simulink model "Battery_TempPredUsingNN_PhysicsModel"  (R2020b)
settings: Solver=ode1be  StartTime=0.0  StopTime=4000  FixedStep=1  MaxStep=5e-2  RelTol=1e-3  AbsTol=1e-3
PreLoadFcn:
  | Battery_TempPredUsingNN_PhysicsModel_ini
undefined symbols (not defined in the file): ambient, Flowrate_vec, FlwR, FlwT
libraries: nesl_utility x19, fl_lib x9, batteryModule_lib x4
Description:
  | Battery Pack Plant Model For Training Neural Network
settings Model: Creator=The MathWorks, Inc.  LastModifiedBy=vikrants
settings SolverCC: AutoScaleAbsTol=off  ZeroCrossAlgorithm=Adaptive
settings DataIOCC: ReturnWorkspaceOutputs=off
settings DebuggingCC: IgnoredZcDiagnostic=none  SymbolicDimsDataTypeCodeGenerationDiagnostic=none
settings SFSimCC: CustomCodeUndefinedFunction=UseInterfaceOnly
settings SimscapeCC: SimscapeLogType=all  SimscapeLogSimulationStatistics=on  SimscapeLogName=simlog_Battery_TempPredUsingNN_PhysicsModel  SimscapeLogDataHistory=250000

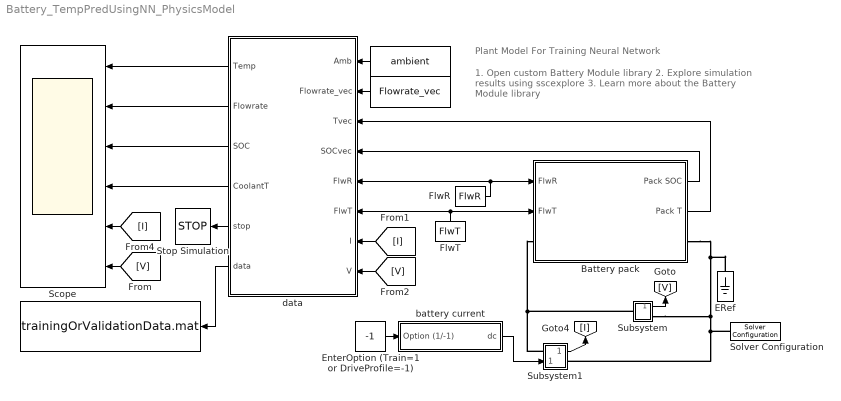
== system Battery_TempPredUsingNN_PhysicsModel ==
  note: Plant Model For Training Neural Network
  note: 1. Open custom Battery Module library
      | 2. Explore simulation results using sscexplore
      | 3. Learn more about the Battery Module library
  " " : ToFile  Filename=trainingOrValidationData.mat  MatrixName=validate_X  SaveFormat=Timeseries
  "    " : Constant  Value=Flowrate_vec
  "       " : Constant  Value=ambient
  Battery pack : Subsystem
      mask Display: image('Battery_Management_System_icon.png'); % Use "Edit Image" on toolstrip to change.
  "ERef " : fl_lib/Electrical/Electrical Elements/Electrical Reference
  EnterOption (Train=1 or DriveProfile=-1) : Constant  Value=-1
  FlwR : Constant  Value=FlwR
  FlwT : Constant  Value=FlwT
  Scope : Scope  NumInputPorts=6
  Solver Configuration : nesl_utility/Solver Configuration  PhysicalDomain=network_engine_domain  SubClassName=solver  LeftPortType=input  RightPortType=generic  Tones=[]  Harmonics=[]  SimulateNoise=off  Profile=off  UseLocalSampling=off  EnableSwitchedLinearOptims=on  FrequencyDomain=off  UseCCode=off  RelTol=0.001  AbsTol=1e-06  MinStep=1e-09  ToWorkspace=off  RevertToSquareIcSolve=off  NumHomotopyIterations=100  PhasorMode=off  PhasorModeNumHarmonics=1  DoDC=off  ResidualTolerance=1e-09  UseLocalSolver=on  LocalSolverChoice=NE_BACKWARD_EULER_ADVANCER  LocalSolverSampleTime=1  DoFixedCost=on  MaxNonlinIter=3  MaxModeIter=2  ComputeImpulses=off  ImpulseIterations=1  LinearAlgebra=auto  EquationFormulation=NE_TIME_EF  DelaysMemoryBudget=1024  AutomaticFiltering=on  FilteringTimeConstant=0.001  PartitionStorageMethod=AS_NEEDED  PartitionMemoryBudget=1024  PartitionMethod=ROBUST
      settings: SourceProductBaseCode=PW,SS
  Stop Simulation : Stop
  Subsystem : Subsystem
  Subsystem1 : Subsystem
      settings: PortSchema="{\"entries\":[{\"content\":{\"sides\":[{\"content\":{\"connectorIds\":[\"LConn1\",\"In1\"]},\"type\":\"ConnectorPlacement.EquallySpacedRectSide\",\"uuid\":\"67d2af16-eb6a-4131-a21a-c97dc5606bfb\"},{\"content\":{\"connectorIds\":[\"Out1\",\"RConn1\"],\"side\":\"RIGHT\"},\"type\":\"ConnectorPlacement.EquallySpacedRectSide\",\"uuid\":\"35a4b5c9-72e5-421e-bb7c-ed2a1ed376d5\"},{\"content\":{\"connectorIds\":[],\"side\":\"TOP\"},\"type\":\"ConnectorPlacement.EquallySpacedRectSide\",\"uuid\":\"8dbff2ba-7191-4b7c-8c3d-553f583a3f33\"},{\"content\":{\"connectorIds\":[],\"side\":\"HIDDEN\"},\"type\":\"ConnectorPlacement.EquallySpacedRectSide\",\"uuid\":\"d4ede02e-0aa1-49c8-8ab9-b8bb5b8f4755\"}]},\"type\":\"ConnectorPlacement.EquallySpacedConnector\",\"uuid\":\"f2085621-9cc2-4a00-8d4f-41f8dda0152d\"}],\"packageUris\":[\"http://schema.mathworks.com/mf0/Connector/R2020b\"],\"version\":\"1.0\"}"
  battery current : Subsystem
  data : Subsystem
  wires:
  Battery pack/2(Pack T) -> data/3(Tvec)
  Battery pack/1(Pack SOC) -> data/4(SOCvec)
  "    "/1 -> data/2(Flowrate_vec)
  "       "/1 -> data/1(Amb)
  [I] -> Scope/5
  data/3(SOC) -> Scope/3
  data/2(Flowrate) -> Scope/2
  FlwT/1 -> data/6(FlwT), Battery pack/2(FlwT)
  data/4(CoolantT) -> Scope/4
  [V] -> Scope/6
  [I] -> data/7(I)
  data/5(stop) -> Stop Simulation/1
  data/6(data) -> " "/1
  [V] -> data/8(V)
  data/1(Temp) -> Scope/1
  FlwR/1 -> Battery pack/1(FlwR), data/5(FlwR)
  Subsystem/1("   ") -> [V]
  Subsystem1/1("   ") -> [I]
  EnterOption (Train=1 or DriveProfile=-1)/1 -> battery current/1(Option (1/-1))
  battery current/1(dc) -> Subsystem1/1(dc)
  connections:
  Battery pack/RConn1 -- "ERef "/LConn1 -- Solver Configuration/RConn1 -- Subsystem1/RConn1 -- Subsystem/RConn1
  Subsystem/LConn1 -- Subsystem1/LConn1 -- Battery pack/LConn1

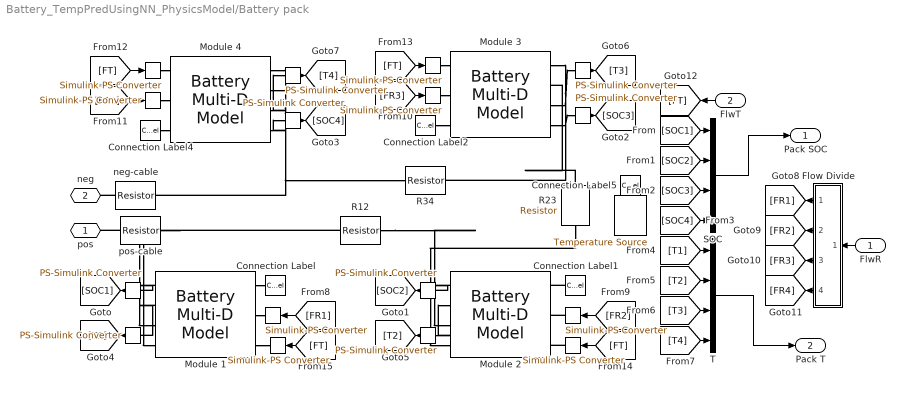
== system Battery_TempPredUsingNN_PhysicsModel/Battery pack ==
  FlwR : Inport
  FlwT : Inport  Port=2
  " " : nesl_utility/PS-Simulink Converter  PhysicalDomain=network_engine_domain  SubClassName=ps_output  LeftPortType=input  RightPortType=output  PseudoPeriodic=off  Frequencies=[]  Unit=inherit  AffineConversion=off
      settings: SourceProductBaseCode=PW,SS
  "  " : nesl_utility/PS-Simulink Converter  PhysicalDomain=network_engine_domain  SubClassName=ps_output  LeftPortType=input  RightPortType=output  PseudoPeriodic=off  Frequencies=[]  Unit=inherit  AffineConversion=off
      settings: SourceProductBaseCode=PW,SS
  "   " : nesl_utility/PS-Simulink Converter  PhysicalDomain=network_engine_domain  SubClassName=ps_output  LeftPortType=input  RightPortType=output  PseudoPeriodic=off  Frequencies=[]  Unit=inherit  AffineConversion=off
      settings: SourceProductBaseCode=PW,SS
  "    " : nesl_utility/Simulink-PS Converter  PhysicalDomain=network_engine_domain  SubClassName=ps_input  LeftPortType=input  RightPortType=output  PseudoPeriodic=off  Frequencies=[]  NoiseDistribution=none  NoiseParameters=[]  Unit=1  AffineConversion=off  FilteringAndDerivatives=filter  SimscapeFilterOrder=1  InputFilterTimeConstant=0.01  UdotUserProvided=0
      settings: SourceProductBaseCode=PW,SS
  "     " : fl_lib/Thermal/Thermal Sources/Temperature Source  temperature=ambient K
  "      " : nesl_utility/PS-Simulink Converter  PhysicalDomain=network_engine_domain  SubClassName=ps_output  LeftPortType=input  RightPortType=output  PseudoPeriodic=off  Frequencies=[]  Unit=inherit  AffineConversion=off
      settings: SourceProductBaseCode=PW,SS
  "       " : nesl_utility/Simulink-PS Converter  PhysicalDomain=network_engine_domain  SubClassName=ps_input  LeftPortType=input  RightPortType=output  PseudoPeriodic=off  Frequencies=[]  NoiseDistribution=none  NoiseParameters=[]  Unit=1  AffineConversion=off  FilteringAndDerivatives=filter  SimscapeFilterOrder=1  InputFilterTimeConstant=0.01  UdotUserProvided=0
      settings: SourceProductBaseCode=PW,SS
  "         " : nesl_utility/PS-Simulink Converter  PhysicalDomain=network_engine_domain  SubClassName=ps_output  LeftPortType=input  RightPortType=output  PseudoPeriodic=off  Frequencies=[]  Unit=inherit  AffineConversion=off
      settings: SourceProductBaseCode=PW,SS
  "          " : nesl_utility/PS-Simulink Converter  PhysicalDomain=network_engine_domain  SubClassName=ps_output  LeftPortType=input  RightPortType=output  PseudoPeriodic=off  Frequencies=[]  Unit=inherit  AffineConversion=off
      settings: SourceProductBaseCode=PW,SS
  "           " : nesl_utility/Simulink-PS Converter  PhysicalDomain=network_engine_domain  SubClassName=ps_input  LeftPortType=input  RightPortType=output  PseudoPeriodic=off  Frequencies=[]  NoiseDistribution=none  NoiseParameters=[]  Unit=1  AffineConversion=off  FilteringAndDerivatives=filter  SimscapeFilterOrder=1  InputFilterTimeConstant=0.01  UdotUserProvided=0
      settings: SourceProductBaseCode=PW,SS
  "            " : nesl_utility/PS-Simulink Converter  PhysicalDomain=network_engine_domain  SubClassName=ps_output  LeftPortType=input  RightPortType=output  PseudoPeriodic=off  Frequencies=[]  Unit=inherit  AffineConversion=off
      settings: SourceProductBaseCode=PW,SS
  "              " : nesl_utility/Simulink-PS Converter  PhysicalDomain=network_engine_domain  SubClassName=ps_input  LeftPortType=input  RightPortType=output  PseudoPeriodic=off  Frequencies=[]  NoiseDistribution=none  NoiseParameters=[]  Unit=1  AffineConversion=off  FilteringAndDerivatives=filter  SimscapeFilterOrder=1  InputFilterTimeConstant=0.01  UdotUserProvided=0
      settings: SourceProductBaseCode=PW,SS
  "               " : nesl_utility/Simulink-PS Converter  PhysicalDomain=network_engine_domain  SubClassName=ps_input  LeftPortType=input  RightPortType=output  PseudoPeriodic=off  Frequencies=[]  NoiseDistribution=none  NoiseParameters=[]  Unit=1  AffineConversion=off  FilteringAndDerivatives=filter  SimscapeFilterOrder=1  InputFilterTimeConstant=0.01  UdotUserProvided=0
      settings: SourceProductBaseCode=PW,SS
  "                      " : nesl_utility/Simulink-PS Converter  PhysicalDomain=network_engine_domain  SubClassName=ps_input  LeftPortType=input  RightPortType=output  PseudoPeriodic=off  Frequencies=[]  NoiseDistribution=none  NoiseParameters=[]  Unit=1  AffineConversion=off  FilteringAndDerivatives=filter  SimscapeFilterOrder=1  InputFilterTimeConstant=0.01  UdotUserProvided=0
      settings: SourceProductBaseCode=PW,SS
  "                                      " : nesl_utility/PS-Simulink Converter  PhysicalDomain=network_engine_domain  SubClassName=ps_output  LeftPortType=input  RightPortType=output  PseudoPeriodic=off  Frequencies=[]  Unit=inherit  AffineConversion=off
      settings: SourceProductBaseCode=PW,SS
  "                                           " : nesl_utility/Simulink-PS Converter  PhysicalDomain=network_engine_domain  SubClassName=ps_input  LeftPortType=input  RightPortType=output  PseudoPeriodic=off  Frequencies=[]  NoiseDistribution=none  NoiseParameters=[]  Unit=1  AffineConversion=off  FilteringAndDerivatives=filter  SimscapeFilterOrder=1  InputFilterTimeConstant=0.01  UdotUserProvided=0
      settings: SourceProductBaseCode=PW,SS
  "                                                  " : nesl_utility/Simulink-PS Converter  PhysicalDomain=network_engine_domain  SubClassName=ps_input  LeftPortType=input  RightPortType=output  PseudoPeriodic=off  Frequencies=[]  NoiseDistribution=none  NoiseParameters=[]  Unit=1  AffineConversion=off  FilteringAndDerivatives=filter  SimscapeFilterOrder=1  InputFilterTimeConstant=0.01  UdotUserProvided=0
      settings: SourceProductBaseCode=PW,SS
  "                        Flow Divide" : Subsystem
  Connection Label{,1..2,4..5} (5 alike) : ConnectionLabel  Label=Amb
  Module 1 : batteryModule_lib/Battery Multi-D Model  modelComplexity=batteryModule.batteryAbstractionLevel.detailed  thermalManagement=batteryModule.batteryCoolingSystem.thermalPort  thermal_moduleBottom=batteryModule.batteryThermalPortSelection.thermalLUT  thermal_moduleTop=batteryModule.batteryThermalPortSelection.convectionBC  thermal_moduleLeft=batteryModule.batteryThermalPortSelection.convectionBC  thermal_moduleRight=batteryModule.batteryThermalPortSelection.convectionBC  thermal_modulePos=batteryModule.batteryThermalPortSelection.convectionBC  thermal_moduleNeg=batteryModule.batteryThermalPortSelection.convectionBC  Ns=Ns  Np=Np  cellTypeSelection=batteryModule.batteryTypeSelection.pouch  cellHeight=cell_H m  cellWidth=cell_W m  cellThickness=cell_T m  cellDiameter=0.018 m  cellCylinLine=3  moduleExternalR=Rext Ohm  LUTpointsTemp=T_vec K  LUTpointsSOC=SOC_vec  cellAHvector=AH_vec hr*A  moduleCellAHpercentVar=AhrVar  cellThermalMass=MdotCp J/K  cellThermalCond=K_cell W/(m*K)  cellThermalCond_inPlane=K_cell W/(m*K)  cellHeatTrCoeff=1 W/(m^2 * K)  htc_bottom=1 W/(m^2 * K)  htc_top=h_cell W/(m^2 * K)  htc_right=h_cell W/(m^2 * K)  htc_left=h_cell W/(m^2 * K)  htc_pos=h_cell W/(m^2 * K)  htc_neg=h_cell W/(m^2 * K)  cellTemp=cellT_ini K  cellSOC=cellSOC_ini  LUTpointsFlowrate_b=Flowrate_vec kg/s  LUTpointsTemp_b=T_vec K  LUTpointsFlowrate_t=[.01, .02, .03, .04, .05, .06] kg/s  LUTpointsTemp_t=[273.15, 298.15, 323.15] K  LUTpointsFlowrate_r=[.01, .02, .03, .04, .05, .06] kg/s  LUTpointsTemp_r=[273.15, 298.15, 323.15] K  LUTpointsFlowrate_l=[.01, .02, .03, .04, .05, .06] kg/s  LUTpointsTemp_l=[273.15, 298.15, 323.15] K  LUTpointsFlowrate_p=[.01, .02, .03, .04, .05, .06] kg/s  LUTpointsTemp_p=[273.15, 298.15, 323.15] K  LUTpointsFlowrate_n=[.01, .02, .03, .04, .05, .06] kg/s  LUTpointsTemp_n=[273.15, 298.15, 323.15] K  moduleCooling_b=coolantQ W/K  moduleCooling_t=zeros(3, 6, 10) W/K  moduleCooling_r=zeros(3, 6, 10) W/K  moduleCooling_l=zeros(3, 6, 10) W/K  moduleCooling_p=zeros(3, 6, 10) W/K  moduleCooling_n=zeros(3, 6, 10) W/K  moduleExtHeat=extHeat W  moduleCellBalancing=batteryModule.batteryCellBalancing.none  moduleCellVoltages=batteryModule.batteryCellVoltages.no  passiveShuntR=50 Ohm  passiveSWclosedR=0.01 Ohm  passiveSWopenCond=1e-8 1/Ohm  passiveSWthreshold=0.5  prm_dir=ee.enum.battery.prm_dir.noCurrentDirectionality  V0_mat=V0_mat V  R0_mat=R0_mat Ohm  R0_dis_mat=[.03, .015, .002; .04, .017, .008; .039, .012, .006; .027, .013, .021] Ohm  R0_ch_mat=[.03, .015, .002; .04, .017, .008; .039, .012, .006; .027, .013, .021] Ohm  moduleCellR0PercentVar=R0Var  prm_leak=ee.enum.battery.prm_leak.disabled  Rleak_vec=[8000, 7000, 6000] Ohm  moduleCellLeakPercentVar=ones(1, 10)  extrapolation_option=ee.enum.extrapolation.nearest  prm_dyn=ee.enum.battery.prm_dyn.off  R1_mat=[.089, .076, .01; .042, .022, .099; .019, .007, .002; .051, .043, .029] Ohm  tau1_mat=[44, 148, 235; 93, 110, 1000; 19, 27, 133; .5, 22, 3] s  R2_mat=[.014, .382, .407; .028, .006, .007; .014, .007, .006; .333, .956, .912] Ohm  tau2_mat=[1, 44, 5644; 11, 24, 506; 2, 14, 330; 3310, 13419, 30216] s  R3_mat=[.014, .382, .407; .028, .006, .007; .014, .007, .006; .333, .956, .912] Ohm  tau3_mat=[1, 44, 5644; 11, 24, 506; 2, 14, 330; 3310, 13419, 30216] s  R4_mat=[.014, .382, .407; .028, .006, .007; .014, .007, .006; .333, .956, .912] Ohm  tau4_mat=[1, 44, 5644; 11, 24, 506; 2, 14, 330; 3310, 13419, 30216] s  R5_mat=[.014, .382, .407; .028, .006, .007; .014, .007, .006; .333, .956, .912] Ohm  tau5_mat=[1, 44, 5644; 11, 24, 506; 2, 14, 330; 3310, 13419, 30216] s  prm_fade=ee.enum.battery.prm_fade.equations  N0=Ndisc  dV0=delV0  dR0=delR0  dAH=delAH  dRleak=0  dR1=0  dR2=0  dR3=0  dR4=0  dR5=0  N0vec=[100, 200, 300]  Tfadevec=[298.15, 323.15] K  dV0vec=[0, 0, 0]  dR0vec=[0, 0, 0]  dAHvec=[0, 0, 0]  dRleakvec=[0, 0, 0]  dR1vec=[0, 0, 0]  dR2vec=[0, 0, 0]  dR3vec=[0, 0, 0]  dR4vec=[0, 0, 0]  dR5vec=[0, 0, 0]  dV0mat=[0, 0; 0, 0; 0, 0]  dR0mat=[0, 0; 0, 0; 0, 0]  dAHmat=[0, 0; 0, 0; 0, 0]  dRleakmat=[0, 0; 0, 0; 0, 0]  dR1mat=[0, 0; 0, 0; 0, 0]  dR2mat=[0, 0; 0, 0; 0, 0]  dR3mat=[0, 0; 0, 0; 0, 0]  dR4mat=[0, 0; 0, 0; 0, 0]  dR5mat=[0, 0; 0, 0; 0, 0]
      settings: InternalSimscapePortConfiguration="{\"Bottom\":[],\"Left\":[{\"id\":\"outputCellSOC\",\"label\":\"SOC\",\"type\":\"output\"},{\"id\":\"outputCellTemp\",\"label\":\"Temp\",\"type\":\"output\"}],\"Right\":[{\"id\":\"H\",\"label\":\"Amb\",\"type\":\"foundation.thermal.thermal\"},{\"id\":\"frac_b\",\"label\":\"FlwR\",\"type\":\"input\"},{\"id\":\"delT_b\",\"label\":\"FlwT\",\"type\":\"input\"}],\"Top\":[{\"id\":\"p\",\"label\":\"pos\",\"type\":\"foundation.electrical.electrical\"},{\"id\":\"n\",\"label\":\"neg\",\"type\":\"foundation.electrical.electrical\"}]}"
  Module 2 : batteryModule_lib/Battery Multi-D Model  modelComplexity=batteryModule.batteryAbstractionLevel.detailed  thermalManagement=batteryModule.batteryCoolingSystem.thermalPort  thermal_moduleBottom=batteryModule.batteryThermalPortSelection.thermalLUT  thermal_moduleTop=batteryModule.batteryThermalPortSelection.convectionBC  thermal_moduleLeft=batteryModule.batteryThermalPortSelection.convectionBC  thermal_moduleRight=batteryModule.batteryThermalPortSelection.convectionBC  thermal_modulePos=batteryModule.batteryThermalPortSelection.convectionBC  thermal_moduleNeg=batteryModule.batteryThermalPortSelection.convectionBC  Ns=Ns  Np=Np  cellTypeSelection=batteryModule.batteryTypeSelection.pouch  cellHeight=cell_H m  cellWidth=cell_W m  cellThickness=cell_T m  cellDiameter=0.018 m  cellCylinLine=3  moduleExternalR=Rext Ohm  LUTpointsTemp=T_vec K  LUTpointsSOC=SOC_vec  cellAHvector=AH_vec hr*A  moduleCellAHpercentVar=AhrVar  cellThermalMass=MdotCp J/K  cellThermalCond=K_cell W/(m*K)  cellThermalCond_inPlane=K_cell W/(m*K)  cellHeatTrCoeff=1 W/(m^2 * K)  htc_bottom=1 W/(m^2 * K)  htc_top=h_cell W/(m^2 * K)  htc_right=h_cell W/(m^2 * K)  htc_left=h_cell W/(m^2 * K)  htc_pos=h_cell W/(m^2 * K)  htc_neg=h_cell W/(m^2 * K)  cellTemp=cellT_ini K  cellSOC=cellSOC_ini  LUTpointsFlowrate_b=Flowrate_vec kg/s  LUTpointsTemp_b=T_vec K  LUTpointsFlowrate_t=[.01, .02, .03, .04, .05, .06] kg/s  LUTpointsTemp_t=[273.15, 298.15, 323.15] K  LUTpointsFlowrate_r=[.01, .02, .03, .04, .05, .06] kg/s  LUTpointsTemp_r=[273.15, 298.15, 323.15] K  LUTpointsFlowrate_l=[.01, .02, .03, .04, .05, .06] kg/s  LUTpointsTemp_l=[273.15, 298.15, 323.15] K  LUTpointsFlowrate_p=[.01, .02, .03, .04, .05, .06] kg/s  LUTpointsTemp_p=[273.15, 298.15, 323.15] K  LUTpointsFlowrate_n=[.01, .02, .03, .04, .05, .06] kg/s  LUTpointsTemp_n=[273.15, 298.15, 323.15] K  moduleCooling_b=coolantQ W/K  moduleCooling_t=zeros(3, 6, 10) W/K  moduleCooling_r=zeros(3, 6, 10) W/K  moduleCooling_l=zeros(3, 6, 10) W/K  moduleCooling_p=zeros(3, 6, 10) W/K  moduleCooling_n=zeros(3, 6, 10) W/K  moduleExtHeat=extHeat W  moduleCellBalancing=batteryModule.batteryCellBalancing.none  moduleCellVoltages=batteryModule.batteryCellVoltages.no  passiveShuntR=50 Ohm  passiveSWclosedR=0.01 Ohm  passiveSWopenCond=1e-8 1/Ohm  passiveSWthreshold=0.5  prm_dir=ee.enum.battery.prm_dir.noCurrentDirectionality  V0_mat=V0_mat V  R0_mat=R0_mat Ohm  R0_dis_mat=[.03, .015, .002; .04, .017, .008; .039, .012, .006; .027, .013, .021] Ohm  R0_ch_mat=[.03, .015, .002; .04, .017, .008; .039, .012, .006; .027, .013, .021] Ohm  moduleCellR0PercentVar=R0Var  prm_leak=ee.enum.battery.prm_leak.disabled  Rleak_vec=[8000, 7000, 6000] Ohm  moduleCellLeakPercentVar=ones(1, 10)  extrapolation_option=ee.enum.extrapolation.nearest  prm_dyn=ee.enum.battery.prm_dyn.off  R1_mat=[.089, .076, .01; .042, .022, .099; .019, .007, .002; .051, .043, .029] Ohm  tau1_mat=[44, 148, 235; 93, 110, 1000; 19, 27, 133; .5, 22, 3] s  R2_mat=[.014, .382, .407; .028, .006, .007; .014, .007, .006; .333, .956, .912] Ohm  tau2_mat=[1, 44, 5644; 11, 24, 506; 2, 14, 330; 3310, 13419, 30216] s  R3_mat=[.014, .382, .407; .028, .006, .007; .014, .007, .006; .333, .956, .912] Ohm  tau3_mat=[1, 44, 5644; 11, 24, 506; 2, 14, 330; 3310, 13419, 30216] s  R4_mat=[.014, .382, .407; .028, .006, .007; .014, .007, .006; .333, .956, .912] Ohm  tau4_mat=[1, 44, 5644; 11, 24, 506; 2, 14, 330; 3310, 13419, 30216] s  R5_mat=[.014, .382, .407; .028, .006, .007; .014, .007, .006; .333, .956, .912] Ohm  tau5_mat=[1, 44, 5644; 11, 24, 506; 2, 14, 330; 3310, 13419, 30216] s  prm_fade=ee.enum.battery.prm_fade.equations  N0=Ndisc  dV0=delV0  dR0=delR0  dAH=delAH  dRleak=0  dR1=0  dR2=0  dR3=0  dR4=0  dR5=0  N0vec=[100, 200, 300]  Tfadevec=[298.15, 323.15] K  dV0vec=[0, 0, 0]  dR0vec=[0, 0, 0]  dAHvec=[0, 0, 0]  dRleakvec=[0, 0, 0]  dR1vec=[0, 0, 0]  dR2vec=[0, 0, 0]  dR3vec=[0, 0, 0]  dR4vec=[0, 0, 0]  dR5vec=[0, 0, 0]  dV0mat=[0, 0; 0, 0; 0, 0]  dR0mat=[0, 0; 0, 0; 0, 0]  dAHmat=[0, 0; 0, 0; 0, 0]  dRleakmat=[0, 0; 0, 0; 0, 0]  dR1mat=[0, 0; 0, 0; 0, 0]  dR2mat=[0, 0; 0, 0; 0, 0]  dR3mat=[0, 0; 0, 0; 0, 0]  dR4mat=[0, 0; 0, 0; 0, 0]  dR5mat=[0, 0; 0, 0; 0, 0]
      settings: InternalSimscapePortConfiguration="{\"Bottom\":[],\"Left\":[{\"id\":\"outputCellSOC\",\"label\":\"SOC\",\"type\":\"output\"},{\"id\":\"outputCellTemp\",\"label\":\"Temp\",\"type\":\"output\"}],\"Right\":[{\"id\":\"H\",\"label\":\"Amb\",\"type\":\"foundation.thermal.thermal\"},{\"id\":\"frac_b\",\"label\":\"FlwR\",\"type\":\"input\"},{\"id\":\"delT_b\",\"label\":\"FlwT\",\"type\":\"input\"}],\"Top\":[{\"id\":\"p\",\"label\":\"pos\",\"type\":\"foundation.electrical.electrical\"},{\"id\":\"n\",\"label\":\"neg\",\"type\":\"foundation.electrical.electrical\"}]}"
  Module 3 : batteryModule_lib/Battery Multi-D Model  modelComplexity=batteryModule.batteryAbstractionLevel.detailed  thermalManagement=batteryModule.batteryCoolingSystem.thermalPort  thermal_moduleBottom=batteryModule.batteryThermalPortSelection.thermalLUT  thermal_moduleTop=batteryModule.batteryThermalPortSelection.convectionBC  thermal_moduleLeft=batteryModule.batteryThermalPortSelection.convectionBC  thermal_moduleRight=batteryModule.batteryThermalPortSelection.convectionBC  thermal_modulePos=batteryModule.batteryThermalPortSelection.convectionBC  thermal_moduleNeg=batteryModule.batteryThermalPortSelection.convectionBC  Ns=Ns  Np=Np  cellTypeSelection=batteryModule.batteryTypeSelection.pouch  cellHeight=cell_H m  cellWidth=cell_W m  cellThickness=cell_T m  cellDiameter=0.018 m  cellCylinLine=3  moduleExternalR=Rext Ohm  LUTpointsTemp=T_vec K  LUTpointsSOC=SOC_vec  cellAHvector=AH_vec hr*A  moduleCellAHpercentVar=AhrVar  cellThermalMass=MdotCp J/K  cellThermalCond=K_cell W/(m*K)  cellThermalCond_inPlane=K_cell W/(m*K)  cellHeatTrCoeff=1 W/(m^2 * K)  htc_bottom=1 W/(m^2 * K)  htc_top=h_cell W/(m^2 * K)  htc_right=h_cell W/(m^2 * K)  htc_left=h_cell W/(m^2 * K)  htc_pos=h_cell W/(m^2 * K)  htc_neg=h_cell W/(m^2 * K)  cellTemp=cellT_ini K  cellSOC=cellSOC_ini  LUTpointsFlowrate_b=Flowrate_vec kg/s  LUTpointsTemp_b=T_vec K  LUTpointsFlowrate_t=[.01, .02, .03, .04, .05, .06] kg/s  LUTpointsTemp_t=[273.15, 298.15, 323.15] K  LUTpointsFlowrate_r=[.01, .02, .03, .04, .05, .06] kg/s  LUTpointsTemp_r=[273.15, 298.15, 323.15] K  LUTpointsFlowrate_l=[.01, .02, .03, .04, .05, .06] kg/s  LUTpointsTemp_l=[273.15, 298.15, 323.15] K  LUTpointsFlowrate_p=[.01, .02, .03, .04, .05, .06] kg/s  LUTpointsTemp_p=[273.15, 298.15, 323.15] K  LUTpointsFlowrate_n=[.01, .02, .03, .04, .05, .06] kg/s  LUTpointsTemp_n=[273.15, 298.15, 323.15] K  moduleCooling_b=coolantQ W/K  moduleCooling_t=zeros(3, 6, 10) W/K  moduleCooling_r=zeros(3, 6, 10) W/K  moduleCooling_l=zeros(3, 6, 10) W/K  moduleCooling_p=zeros(3, 6, 10) W/K  moduleCooling_n=zeros(3, 6, 10) W/K  moduleExtHeat=extHeat W  moduleCellBalancing=batteryModule.batteryCellBalancing.none  moduleCellVoltages=batteryModule.batteryCellVoltages.no  passiveShuntR=50 Ohm  passiveSWclosedR=0.01 Ohm  passiveSWopenCond=1e-8 1/Ohm  passiveSWthreshold=0.5  prm_dir=ee.enum.battery.prm_dir.noCurrentDirectionality  V0_mat=V0_mat V  R0_mat=R0_mat Ohm  R0_dis_mat=[.03, .015, .002; .04, .017, .008; .039, .012, .006; .027, .013, .021] Ohm  R0_ch_mat=[.03, .015, .002; .04, .017, .008; .039, .012, .006; .027, .013, .021] Ohm  moduleCellR0PercentVar=R0Var  prm_leak=ee.enum.battery.prm_leak.disabled  Rleak_vec=[8000, 7000, 6000] Ohm  moduleCellLeakPercentVar=ones(1, 10)  extrapolation_option=ee.enum.extrapolation.nearest  prm_dyn=ee.enum.battery.prm_dyn.off  R1_mat=[.089, .076, .01; .042, .022, .099; .019, .007, .002; .051, .043, .029] Ohm  tau1_mat=[44, 148, 235; 93, 110, 1000; 19, 27, 133; .5, 22, 3] s  R2_mat=[.014, .382, .407; .028, .006, .007; .014, .007, .006; .333, .956, .912] Ohm  tau2_mat=[1, 44, 5644; 11, 24, 506; 2, 14, 330; 3310, 13419, 30216] s  R3_mat=[.014, .382, .407; .028, .006, .007; .014, .007, .006; .333, .956, .912] Ohm  tau3_mat=[1, 44, 5644; 11, 24, 506; 2, 14, 330; 3310, 13419, 30216] s  R4_mat=[.014, .382, .407; .028, .006, .007; .014, .007, .006; .333, .956, .912] Ohm  tau4_mat=[1, 44, 5644; 11, 24, 506; 2, 14, 330; 3310, 13419, 30216] s  R5_mat=[.014, .382, .407; .028, .006, .007; .014, .007, .006; .333, .956, .912] Ohm  tau5_mat=[1, 44, 5644; 11, 24, 506; 2, 14, 330; 3310, 13419, 30216] s  prm_fade=ee.enum.battery.prm_fade.equations  N0=Ndisc  dV0=delV0  dR0=delR0  dAH=delAH  dRleak=0  dR1=0  dR2=0  dR3=0  dR4=0  dR5=0  N0vec=[100, 200, 300]  Tfadevec=[298.15, 323.15] K  dV0vec=[0, 0, 0]  dR0vec=[0, 0, 0]  dAHvec=[0, 0, 0]  dRleakvec=[0, 0, 0]  dR1vec=[0, 0, 0]  dR2vec=[0, 0, 0]  dR3vec=[0, 0, 0]  dR4vec=[0, 0, 0]  dR5vec=[0, 0, 0]  dV0mat=[0, 0; 0, 0; 0, 0]  dR0mat=[0, 0; 0, 0; 0, 0]  dAHmat=[0, 0; 0, 0; 0, 0]  dRleakmat=[0, 0; 0, 0; 0, 0]  dR1mat=[0, 0; 0, 0; 0, 0]  dR2mat=[0, 0; 0, 0; 0, 0]  dR3mat=[0, 0; 0, 0; 0, 0]  dR4mat=[0, 0; 0, 0; 0, 0]  dR5mat=[0, 0; 0, 0; 0, 0]
      settings: InternalSimscapePortConfiguration="{\"Bottom\":[],\"Left\":[{\"id\":\"outputCellSOC\",\"label\":\"SOC\",\"type\":\"output\"},{\"id\":\"outputCellTemp\",\"label\":\"Temp\",\"type\":\"output\"}],\"Right\":[{\"id\":\"H\",\"label\":\"Amb\",\"type\":\"foundation.thermal.thermal\"},{\"id\":\"frac_b\",\"label\":\"FlwR\",\"type\":\"input\"},{\"id\":\"delT_b\",\"label\":\"FlwT\",\"type\":\"input\"}],\"Top\":[{\"id\":\"p\",\"label\":\"pos\",\"type\":\"foundation.electrical.electrical\"},{\"id\":\"n\",\"label\":\"neg\",\"type\":\"foundation.electrical.electrical\"}]}"
  Module 4 : batteryModule_lib/Battery Multi-D Model  modelComplexity=batteryModule.batteryAbstractionLevel.detailed  thermalManagement=batteryModule.batteryCoolingSystem.thermalPort  thermal_moduleBottom=batteryModule.batteryThermalPortSelection.thermalLUT  thermal_moduleTop=batteryModule.batteryThermalPortSelection.convectionBC  thermal_moduleLeft=batteryModule.batteryThermalPortSelection.convectionBC  thermal_moduleRight=batteryModule.batteryThermalPortSelection.convectionBC  thermal_modulePos=batteryModule.batteryThermalPortSelection.convectionBC  thermal_moduleNeg=batteryModule.batteryThermalPortSelection.convectionBC  Ns=Ns4  Np=Np4  cellTypeSelection=batteryModule.batteryTypeSelection.pouch  cellHeight=cell_H m  cellWidth=cell_W m  cellThickness=cell_T m  cellDiameter=0.018 m  cellCylinLine=3  moduleExternalR=Rext4 Ohm  LUTpointsTemp=T_vec K  LUTpointsSOC=SOC_vec  cellAHvector=AH_vec hr*A  moduleCellAHpercentVar=AhrVar4  cellThermalMass=MdotCp J/K  cellThermalCond=K_cell W/(m*K)  cellThermalCond_inPlane=K_cell W/(m*K)  cellHeatTrCoeff=1 W/(m^2 * K)  htc_bottom=1 W/(m^2 * K)  htc_top=h_cell W/(m^2 * K)  htc_right=h_cell W/(m^2 * K)  htc_left=h_cell W/(m^2 * K)  htc_pos=h_cell W/(m^2 * K)  htc_neg=h_cell W/(m^2 * K)  cellTemp=cellT_ini4 K  cellSOC=cellSOC_ini4  LUTpointsFlowrate_b=Flowrate_vec kg/s  LUTpointsTemp_b=T_vec K  LUTpointsFlowrate_t=[.01, .02, .03, .04, .05, .06] kg/s  LUTpointsTemp_t=[273.15, 298.15, 323.15] K  LUTpointsFlowrate_r=[.01, .02, .03, .04, .05, .06] kg/s  LUTpointsTemp_r=[273.15, 298.15, 323.15] K  LUTpointsFlowrate_l=[.01, .02, .03, .04, .05, .06] kg/s  LUTpointsTemp_l=[273.15, 298.15, 323.15] K  LUTpointsFlowrate_p=[.01, .02, .03, .04, .05, .06] kg/s  LUTpointsTemp_p=[273.15, 298.15, 323.15] K  LUTpointsFlowrate_n=[.01, .02, .03, .04, .05, .06] kg/s  LUTpointsTemp_n=[273.15, 298.15, 323.15] K  moduleCooling_b=coolantQ4 W/K  moduleCooling_t=zeros(3, 6, 10) W/K  moduleCooling_r=zeros(3, 6, 10) W/K  moduleCooling_l=zeros(3, 6, 10) W/K  moduleCooling_p=zeros(3, 6, 10) W/K  moduleCooling_n=zeros(3, 6, 10) W/K  moduleExtHeat=extHeat4 W  moduleCellBalancing=batteryModule.batteryCellBalancing.none  moduleCellVoltages=batteryModule.batteryCellVoltages.no  passiveShuntR=50 Ohm  passiveSWclosedR=0.01 Ohm  passiveSWopenCond=1e-8 1/Ohm  passiveSWthreshold=0.5  prm_dir=ee.enum.battery.prm_dir.noCurrentDirectionality  V0_mat=V0_mat V  R0_mat=R0_mat Ohm  R0_dis_mat=[.03, .015, .002; .04, .017, .008; .039, .012, .006; .027, .013, .021] Ohm  R0_ch_mat=[.03, .015, .002; .04, .017, .008; .039, .012, .006; .027, .013, .021] Ohm  moduleCellR0PercentVar=R0Var4  prm_leak=ee.enum.battery.prm_leak.disabled  Rleak_vec=[8000, 7000, 6000] Ohm  moduleCellLeakPercentVar=ones(1, 10)  extrapolation_option=ee.enum.extrapolation.nearest  prm_dyn=ee.enum.battery.prm_dyn.off  R1_mat=[.089, .076, .01; .042, .022, .099; .019, .007, .002; .051, .043, .029] Ohm  tau1_mat=[44, 148, 235; 93, 110, 1000; 19, 27, 133; .5, 22, 3] s  R2_mat=[.014, .382, .407; .028, .006, .007; .014, .007, .006; .333, .956, .912] Ohm  tau2_mat=[1, 44, 5644; 11, 24, 506; 2, 14, 330; 3310, 13419, 30216] s  R3_mat=[.014, .382, .407; .028, .006, .007; .014, .007, .006; .333, .956, .912] Ohm  tau3_mat=[1, 44, 5644; 11, 24, 506; 2, 14, 330; 3310, 13419, 30216] s  R4_mat=[.014, .382, .407; .028, .006, .007; .014, .007, .006; .333, .956, .912] Ohm  tau4_mat=[1, 44, 5644; 11, 24, 506; 2, 14, 330; 3310, 13419, 30216] s  R5_mat=[.014, .382, .407; .028, .006, .007; .014, .007, .006; .333, .956, .912] Ohm  tau5_mat=[1, 44, 5644; 11, 24, 506; 2, 14, 330; 3310, 13419, 30216] s  prm_fade=ee.enum.battery.prm_fade.equations  N0=Ndisc  dV0=delV0  dR0=delR0  dAH=delAH  dRleak=0  dR1=0  dR2=0  dR3=0  dR4=0  dR5=0  N0vec=[100, 200, 300]  Tfadevec=[298.15, 323.15] K  dV0vec=[0, 0, 0]  dR0vec=[0, 0, 0]  dAHvec=[0, 0, 0]  dRleakvec=[0, 0, 0]  dR1vec=[0, 0, 0]  dR2vec=[0, 0, 0]  dR3vec=[0, 0, 0]  dR4vec=[0, 0, 0]  dR5vec=[0, 0, 0]  dV0mat=[0, 0; 0, 0; 0, 0]  dR0mat=[0, 0; 0, 0; 0, 0]  dAHmat=[0, 0; 0, 0; 0, 0]  dRleakmat=[0, 0; 0, 0; 0, 0]  dR1mat=[0, 0; 0, 0; 0, 0]  dR2mat=[0, 0; 0, 0; 0, 0]  dR3mat=[0, 0; 0, 0; 0, 0]  dR4mat=[0, 0; 0, 0; 0, 0]  dR5mat=[0, 0; 0, 0; 0, 0]
      settings: InternalSimscapePortConfiguration="{\"Bottom\":[],\"Left\":[{\"id\":\"outputCellSOC\",\"label\":\"SOC\",\"type\":\"output\"},{\"id\":\"outputCellTemp\",\"label\":\"Temp\",\"type\":\"output\"}],\"Right\":[{\"id\":\"H\",\"label\":\"Amb\",\"type\":\"foundation.thermal.thermal\"},{\"id\":\"frac_b\",\"label\":\"FlwR\",\"type\":\"input\"},{\"id\":\"delT_b\",\"label\":\"FlwT\",\"type\":\"input\"}],\"Top\":[{\"id\":\"p\",\"label\":\"pos\",\"type\":\"foundation.electrical.electrical\"},{\"id\":\"n\",\"label\":\"neg\",\"type\":\"foundation.electrical.electrical\"}]}"
  R12 : fl_lib/Electrical/Electrical Elements/Resistor  R=0.001 Ohm  i_specify=off  i_priority=None  i=0 A  i_nominal_specify=off  i_nominal_unit=A  i_nominal_value=1  v_specify=off  v_priority=None  v=0 V  v_nominal_specify=off  v_nominal_unit=V  v_nominal_value=1
  R23 : fl_lib/Electrical/Electrical Elements/Resistor  R=0.001 Ohm  i_specify=off  i_priority=None  i=0 A  i_nominal_specify=off  i_nominal_unit=A  i_nominal_value=1  v_specify=off  v_priority=None  v=0 V  v_nominal_specify=off  v_nominal_unit=V  v_nominal_value=1
  R34 : fl_lib/Electrical/Electrical Elements/Resistor  R=0.001 Ohm  i_specify=off  i_priority=None  i=0 A  i_nominal_specify=off  i_nominal_unit=A  i_nominal_value=1  v_specify=off  v_priority=None  v=0 V  v_nominal_specify=off  v_nominal_unit=V  v_nominal_value=1
  SOC : Concatenate  NumInputs=4
  T : Concatenate  NumInputs=4
  neg-cable : fl_lib/Electrical/Electrical Elements/Resistor  R=0.001 Ohm  i_specify=off  i_priority=None  i=0 A  i_nominal_specify=off  i_nominal_unit=A  i_nominal_value=1  v_specify=off  v_priority=None  v=0 V  v_nominal_specify=off  v_nominal_unit=V  v_nominal_value=1
  pos-cable : fl_lib/Electrical/Electrical Elements/Resistor  R=0.001 Ohm  i_specify=off  i_priority=None  i=0 A  i_nominal_specify=off  i_nominal_unit=A  i_nominal_value=1  v_specify=off  v_priority=None  v=0 V  v_nominal_specify=off  v_nominal_unit=V  v_nominal_value=1
  pos : PMIOPort  Side=Left
  neg : PMIOPort  Port=2  Side=Right
  Pack SOC : Outport
  Pack T : Outport  Port=2
  wires:
  "  "/1 -> [SOC1]
  "      "/1 -> [SOC2]
  "          "/1 -> [SOC3]
  "            "/1 -> [SOC4]
  [SOC1] -> SOC/1
  [SOC2] -> SOC/2
  [SOC3] -> SOC/3
  [SOC4] -> SOC/4
  [T3] -> T/3
  [T4] -> T/4
  [T2] -> T/2
  [T1] -> T/1
  " "/1 -> [T1]
  "   "/1 -> [T2]
  "         "/1 -> [T3]
  "                                      "/1 -> [T4]
  [FR1] -> "    "/1
  [FR2] -> "       "/1
  [FR3] -> "                      "/1
  [FR4] -> "           "/1
  [FT] -> "               "/1
  [FT] -> "              "/1
  [FT] -> "                                                  "/1
  [FT] -> "                                           "/1
  FlwT/1 -> [FT]
  SOC/1 -> Pack SOC/1
  T/1 -> Pack T/1
  FlwR/1 -> "                        Flow Divide"/1(In1)
  "                        Flow Divide"/1(Out1) -> [FR1]
  "                        Flow Divide"/2(Out2) -> [FR2]
  "                        Flow Divide"/3(Out3) -> [FR3]
  "                        Flow Divide"/4(Out4) -> [FR4]
  connections:
  "              "/RConn1 -- Module 3/RConn3
  "           "/RConn1 -- Module 4/RConn2
  Module 1/LConn2 -- " "/LConn1
  Module 4/LConn1 -- "            "/LConn1
  Module 2/LConn1 -- "      "/LConn1
  "   "/LConn1 -- Module 2/LConn2
  "               "/RConn1 -- Module 4/RConn3
  "                      "/RConn1 -- Module 3/RConn2
  "       "/RConn1 -- Module 2/RConn2
  Module 1/LConn1 -- "  "/LConn1
  Module 3/LConn1 -- "          "/LConn1
  Module 3/LConn2 -- "         "/LConn1
  Module 1/RConn1 -- Connection Label/LConn1
  Connection Label1/LConn1 -- Module 2/RConn1
  Connection Label2/LConn1 -- Module 3/RConn1
  Connection Label4/LConn1 -- Module 4/RConn1
  Connection Label5/LConn1 -- "     "/LConn1
  Module 1/RConn2 -- "    "/RConn1
  "                                                  "/RConn1 -- Module 2/RConn3
  Module 1/RConn3 -- "                                           "/RConn1
  R12/LConn1 -- Module 1/LConn4
  R12/RConn1 -- Module 2/LConn3
  Module 3/LConn4 -- R34/LConn1
  Module 4/LConn3 -- R34/RConn1
  R23/RConn1 -- Module 3/LConn3
  R23/LConn1 -- Module 2/LConn4
  neg-cable/RConn1 -- neg/RConn1
  Module 4/LConn4 -- neg-cable/LConn1
  pos-cable/LConn1 -- pos/RConn1
  pos-cable/RConn1 -- Module 1/LConn3
  Module 4/LConn2 -- "                                      "/LConn1

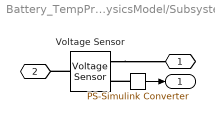
== system Battery_TempPredUsingNN_PhysicsModel/Subsystem ==
  "  " : nesl_utility/PS-Simulink Converter  PhysicalDomain=network_engine_domain  SubClassName=ps_output  LeftPortType=input  RightPortType=output  PseudoPeriodic=off  Frequencies=[]  Unit=inherit  AffineConversion=off
      settings: SourceProductBaseCode=PW,SS
  Voltage Sensor : fl_lib/Electrical/Electrical Sensors/Voltage Sensor
  "    " : PMIOPort  Side=Right
  " " : PMIOPort  Port=2  Side=Left
  "   " : Outport
  wires:
  "  "/1 -> "   "/1
  connections:
  Voltage Sensor/RConn2 -- "    "/RConn1
  "  "/LConn1 -- Voltage Sensor/RConn1
  Voltage Sensor/LConn1 -- " "/RConn1

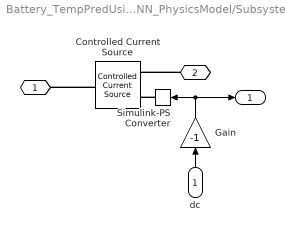
== system Battery_TempPredUsingNN_PhysicsModel/Subsystem1 ==
  dc : Inport
  Controlled Current Source : fl_lib/Electrical/Electrical Sources/Controlled Current Source
  Gain : Gain  Gain=-1
  Simulink-PS Converter : nesl_utility/Simulink-PS Converter  PhysicalDomain=network_engine_domain  SubClassName=ps_input  LeftPortType=input  RightPortType=output  PseudoPeriodic=off  Frequencies=[]  NoiseDistribution=none  NoiseParameters=[]  Unit=A  AffineConversion=off  FilteringAndDerivatives=filter  SimscapeFilterOrder=1  InputFilterTimeConstant=0.01  UdotUserProvided=0
      settings: SourceProductBaseCode=PW,SS
  " " : PMIOPort  Side=Left
  "    " : PMIOPort  Port=2  Side=Right
  "   " : Outport
  wires:
  dc/1 -> Gain/1
  Gain/1 -> "   "/1, Simulink-PS Converter/1
  connections:
  "    "/RConn1 -- Controlled Current Source/RConn2
  Controlled Current Source/LConn1 -- " "/RConn1
  Simulink-PS Converter/RConn1 -- Controlled Current Source/RConn1

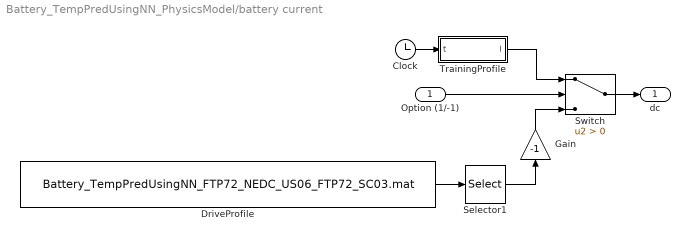
== system Battery_TempPredUsingNN_PhysicsModel/battery current ==
  Option (1/-1) : Inport
  Clock : Clock
  DriveProfile : FromFile  FileName=Battery_TempPredUsingNN_FTP72_NEDC_US06_FTP72_SC03.mat  SampleTime=0
  Gain : Gain  Gain=-1
  Selector1 : Selector  InputPortWidth=5  IndexOptions=Index vector (dialog)  Indices=1  OutputSizes=1
  Switch : Switch  Criteria=u2 > Threshold
  TrainingProfile : MATLAB Function  TreatAsAtomicUnit=on
  dc : Outport
  wires:
  Clock/1 -> TrainingProfile/1(t)
  TrainingProfile/1(I) -> Switch/1
  Switch/1 -> dc/1
  Option (1/-1)/1 -> Switch/2
  DriveProfile/1 -> Selector1/1
  Selector1/1 -> Gain/1
  Gain/1 -> Switch/3

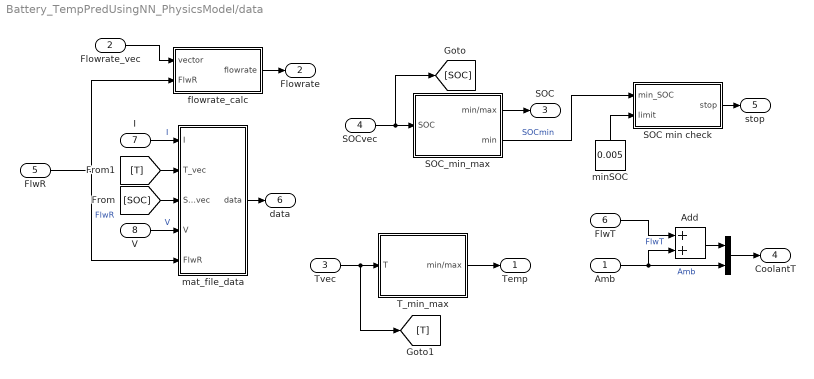
== system Battery_TempPredUsingNN_PhysicsModel/data ==
  Amb : Inport
  Flowrate_vec : Inport  Port=2
  Tvec : Inport  Port=3
  SOCvec : Inport  Port=4
  FlwR : Inport  Port=5
  FlwT : Inport  Port=6
  I : Inport  Port=7
  V : Inport  Port=8
  " " : Concatenate
  Add : Sum
  SOC min check : Subsystem
  SOC_min_max : Subsystem
  T_min_max : Subsystem
  flowrate_calc : Subsystem
  mat_file_data : Subsystem
  minSOC : Constant  Value=0.005
  Temp : Outport
  Flowrate : Outport  Port=2
  SOC : Outport  Port=3
  CoolantT : Outport  Port=4
  stop : Outport  Port=5
  data : Outport  Port=6
  wires:
  SOCvec/1 -> [SOC], SOC_min_max/1(SOC)
  SOC_min_max/1(min/max) -> SOC/1
  T_min_max/1(min/max) -> Temp/1
  Tvec/1 -> [T], T_min_max/1(T)
  FlwT/1 -> Add/1  "FlwT"
  Amb/1 -> " "/2, Add/2  "Amb"
  FlwR/1 -> mat_file_data/5(FlwR), flowrate_calc/2(FlwR)  "FlwR"
  Add/1 -> " "/1
  " "/1 -> CoolantT/1
  SOC_min_max/2(min) -> SOC min check/1(min_SOC)  "SOCmin"
  SOC min check/1(stop) -> stop/1
  I/1 -> mat_file_data/1(I)  "I"
  V/1 -> mat_file_data/4(V)  "V"
  mat_file_data/1(data) -> data/1
  Flowrate_vec/1 -> flowrate_calc/1(vector)
  flowrate_calc/1(flowrate) -> Flowrate/1
  [SOC] -> mat_file_data/3(SOC_vec)
  [T] -> mat_file_data/2(T_vec)
  minSOC/1 -> SOC min check/2(limit)

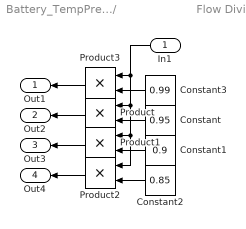
== system Battery_TempPredUsingNN_PhysicsModel/Battery pack/                        Flow Divide ==
  In1 : Inport
  Constant : Constant  Value=0.95
  Constant1 : Constant  Value=0.9
  Constant2 : Constant  Value=0.85
  Constant3 : Constant  Value=0.99
  Product{,1..3} (4 alike) : Product
  Out1 : Outport
  Out2 : Outport  Port=2
  Out3 : Outport  Port=3
  Out4 : Outport  Port=4
  wires:
  Constant1/1 -> Product1/2
  Constant/1 -> Product/2
  Product/1 -> Out2/1
  In1/1 -> Product2/1, Product1/1, Product/1, Product3/1
  Constant3/1 -> Product3/2
  Product1/1 -> Out3/1
  Constant2/1 -> Product2/2
  Product3/1 -> Out1/1
  Product2/1 -> Out4/1

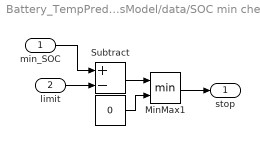
== system Battery_TempPredUsingNN_PhysicsModel/data/SOC min check ==
  min_SOC : Inport
  limit : Inport  Port=2
  "   " : Constant  Value=0
  MinMax1 : MinMax  Inputs=2  ZeroCross=off
  Subtract : Sum  Inputs=+-
  stop : Outport
  wires:
  "   "/1 -> MinMax1/2
  Subtract/1 -> MinMax1/1
  min_SOC/1 -> Subtract/1
  MinMax1/1 -> stop/1
  limit/1 -> Subtract/2

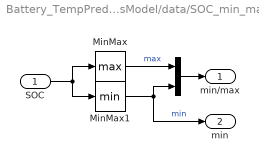
== system Battery_TempPredUsingNN_PhysicsModel/data/SOC_min_max ==
  SOC : Inport
  " " : Concatenate
  MinMax : MinMax  Function=max  ZeroCross=off
  MinMax1 : MinMax  ZeroCross=off
  min/max : Outport
  min : Outport  Port=2
  wires:
  MinMax1/1 -> " "/2, min/1  "min"
  SOC/1 -> MinMax1/1, MinMax/1
  " "/1 -> min/max/1
  MinMax/1 -> " "/1  "max"

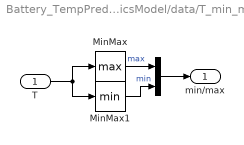
== system Battery_TempPredUsingNN_PhysicsModel/data/T_min_max ==
  T : Inport
  " " : Concatenate
  MinMax : MinMax  Function=max  ZeroCross=off
  MinMax1 : MinMax  ZeroCross=off
  min/max : Outport
  wires:
  MinMax1/1 -> " "/2  "min"
  T/1 -> MinMax1/1, MinMax/1
  " "/1 -> min/max/1
  MinMax/1 -> " "/1  "max"

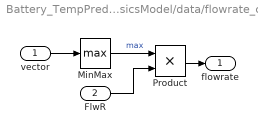
== system Battery_TempPredUsingNN_PhysicsModel/data/flowrate_calc ==
  vector : Inport
  FlwR : Inport  Port=2
  MinMax : MinMax  Function=max  ZeroCross=off
  Product : Product
  flowrate : Outport
  wires:
  Product/1 -> flowrate/1
  MinMax/1 -> Product/1  "max"
  FlwR/1 -> Product/2
  vector/1 -> MinMax/1

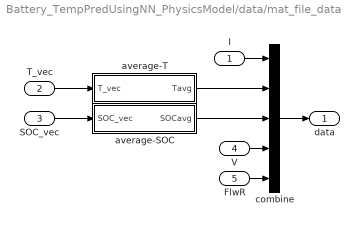
== system Battery_TempPredUsingNN_PhysicsModel/data/mat_file_data ==
  I : Inport
  T_vec : Inport  Port=2
  SOC_vec : Inport  Port=3
  V : Inport  Port=4
  FlwR : Inport  Port=5
  average-SOC : Subsystem
  average-T : Subsystem
  combine : Concatenate  NumInputs=5
  data : Outport
  wires:
  combine/1 -> data/1
  T_vec/1 -> average-T/1(T_vec)
  average-SOC/1(SOCavg) -> combine/3
  I/1 -> combine/1
  SOC_vec/1 -> average-SOC/1(SOC_vec)
  average-T/1(Tavg) -> combine/2
  V/1 -> combine/4
  FlwR/1 -> combine/5

== system Battery_TempPredUsingNN_PhysicsModel/data/mat_file_data/average-SOC ==
  SOC_vec : Inport
  Divide1 : Product  Inputs=*/
  MATLAB Function1 : MATLAB Function  TreatAsAtomicUnit=on
  Sum of Elements1 : Sum  Inputs=+
  SOCavg : Outport
  wires:
  MATLAB Function1/1(y) -> Divide1/2
  Sum of Elements1/1 -> Divide1/1
  Divide1/1 -> SOCavg/1  "SOCavg"
  SOC_vec/1 -> MATLAB Function1/1(u), Sum of Elements1/1

== system Battery_TempPredUsingNN_PhysicsModel/data/mat_file_data/average-T ==
  T_vec : Inport
  Divide : Product  Inputs=*/
  MATLAB Function : MATLAB Function  TreatAsAtomicUnit=on
  Sum of Elements : Sum  Inputs=+
  Tavg : Outport
  wires:
  Sum of Elements/1 -> Divide/1
  MATLAB Function/1(y) -> Divide/2
  Divide/1 -> Tavg/1  "Tavg"
  T_vec/1 -> MATLAB Function/1(u), Sum of Elements/1

== matlab function Battery_TempPredUsingNN_PhysicsModel/data/mat_file_data/average-T/MATLAB Function ==
  data: u input; y output
function y = fcn(u)
y = length(u);
end

== matlab function Battery_TempPredUsingNN_PhysicsModel/battery current/TrainingProfile ==
  data: t input; I output
function I = current(t)
    cap_ahr=18.5*2;  % Parallel unit cell capacity, Np=2
    oneHr=0.98*3600; % seconds
    firstChrDischg_t=oneHr;
    restTime=oneHr;
    t_option_gt_1=firstChrDischg_t+oneHr+2*oneHr/1.5+2*oneHr/2+2*oneHr/2.5+2*oneHr/3+restTime;
    if t<=t_option_gt_1
        % Low to High C rate cycling + rest time
        option=2;
    else
        % High to Low C rate cycling
        option=0;
    end
    %
    if option>1
        if t<firstChrDischg_t
            C_rate=1;
            chgDischg=-1;
        elseif t>=firstChrDischg_t && ...
               t<firstChrDischg_t+oneHr
            C_rate=1;
            chgDischg=1;
        elseif t>=firstChrDischg_t+oneHr && ...
               t<firstChrDischg_t+oneHr+oneHr/1.5
            C_rate=1.5;
            chgDischg=-1;
        elseif t>=firstChrDischg_t+oneHr+oneHr/1.5 && ...
               t<firstChrDischg_t+oneHr+2*oneHr/1.5
            C_rate=1.5;
            chgDischg=1;
        elseif t>=firstChrDischg_t+oneHr+2*oneHr/1.5 && ...
               t<firstChrDischg_t+oneHr+2*oneHr/1.5+oneHr/2
            C_rate=2;
            chgDischg=-1;
        elseif t>=firstChrDischg_t+oneHr+2*oneHr/1.5+oneHr/2 && ...
               t<firstChrDischg_t+oneHr+2*oneHr/1.5+2*oneHr/2
            C_rate=2;
            chgDischg=1;
        elseif t>=firstChrDischg_t+oneHr+2*oneHr/1.5+2*oneHr/2 && ...
               t<firstChrDischg_t+oneHr+2*oneHr/1.5+2*oneHr/2+oneHr/2.5
            C_rate=2.5;
            chgDischg=-1;
        elseif t>=firstChrDischg_t+oneHr+2*oneHr/1.5+2*oneHr/2+oneHr/2.5 && ...
               t<firstChrDischg_t+oneHr+2*oneHr/1.5+2*oneHr/2+2*oneHr/2.5
            C_rate=2.5;
            chgDischg=1;
        elseif t>=firstChrDischg_t+oneHr+2*oneHr/1.5+2*oneHr/2+2*oneHr/2.5 && ...
               t<firstChrDischg_t+oneHr+2*oneHr/1.5+2*oneHr/2+2*oneHr/2.5+oneHr/3
            C_rate=3;
            chgDischg=-1;
        elseif t>=firstChrDischg_t+oneHr+2*oneHr/1.5+2*oneHr/2+2*oneHr/2.5+oneHr/3 && ...
               t<firstChrDischg_t+oneHr+2*oneHr/1.5+2*oneHr/2+2*oneHr/2.5+2*oneHr/3
            C_rate=3;
            chgDischg=1;
        else
            C_rate=0.001;
            chgDischg=1;
        end
    else    
        if t<t_option_gt_1+firstChrDischg_t/3
            C_rate=3;
            chgDischg=-1;
        elseif t>=t_option_gt_1+firstChrDischg_t/3 && ...
               t<t_option_gt_1+2*firstChrDischg_t/3
            C_rate=3;
            chgDischg=1;
        elseif t>=t_option_gt_1+2*firstChrDischg_t/3 && ...
               t<t_option_gt_1+2*firstChrDischg_t/3+oneHr/2.5
            C_rate=2.5;
            chgDischg=-1;
        elseif t>=t_option_gt_1+2*firstChrDischg_t/3+oneHr/2.5 && ...
               t<t_option_gt_1+2*firstChrDischg_t/3+2*oneHr/2.5
            C_rate=2.5;
            chgDischg=1;
        elseif t>=t_option_gt_1+2*firstChrDischg_t/3+2*oneHr/2.5 && ...
               t<t_option_gt_1+2*firstChrDischg_t/3+2*oneHr/2.5+oneHr/2
            C_rate=2;
            chgDischg=-1;
        elseif t>=t_option_gt_1+2*firstChrDischg_t/3+2*oneHr/2.5+oneHr/2 && ...
               t<t_option_gt_1+2*firstChrDischg_t/3+2*oneHr/2.5+2*oneHr/2
            C_rate=2;
            chgDischg=1;
        elseif t>=t_option_gt_1+2*firstChrDischg_t/3+2*oneHr/2.5+2*oneHr/2 && ...
               t<t_option_gt_1+2*firstChrDischg_t/3+2*oneHr/2.5+2*oneHr/2+oneHr/1.5
            C_rate=1.5;
            chgDischg=-1;
        elseif t>=t_option_gt_1+2*firstChrDischg_t/3+2*oneHr/2.5+2*oneHr/2+oneHr/1.5 && ...
               t<t_option_gt_1+2*firstChrDischg_t/3+2*oneHr/2.5+2*oneHr/2+2*oneHr/1.5
            C_rate=1.5;
            chgDischg=1;
        elseif t>=t_option_gt_1+2*firstChrDischg_t/3+2*oneHr/2.5+2*oneHr/2+2*oneHr/1.5 && ...
               t<t_option_gt_1+2*firstChrDischg_t/3+2*oneHr/2.5+2*oneHr/2+2*oneHr/1.5+oneHr
            C_rate=1;
            chgDischg=-1;
        elseif t>=t_option_gt_1+2*firstChrDischg_t/3+2*oneHr/2.5+2*oneHr/2+2*oneHr/1.5+oneHr && ...
               t<t_option_gt_1+2*firstChrDischg_t/3+2*oneHr/2.5+2*oneHr/2+2*oneHr/1.5+2*oneHr
            C_rate=1;
            chgDischg=1;
        elseif t>=t_option_gt_1+2*firstChrDischg_t/3+2*oneHr/2.5+2*oneHr/2+2*oneHr/1.5+2*oneHr && ...
               t<t_option_gt_1+2*firstChrDischg_t/3+2*oneHr/2.5+2*oneHr/2+2*oneHr/1.5+2*oneHr+7150
            C_rate=0.5;
            chgDischg=-1;
        elseif t>=t_option_gt_1+2*firstChrDischg_t/3+2*oneHr/2.5+2*oneHr/2+2*oneHr/1.5+2*oneHr+7150 && ...
               t<t_option_gt_1+2*firstChrDischg_t/3+2*oneHr/2.5+2*oneHr/2+2*oneHr/1.5+2*oneHr+2*7150
            C_rate=0.5;
            chgDischg=1;
        else
            C_rate=0.001;
            chgDischg=-1;
        end
    end
    I=(-1)*cap_ahr*chgDischg*C_rate;
end

== matlab function Battery_TempPredUsingNN_PhysicsModel/data/mat_file_data/average-SOC/MATLAB Function1 ==
  data: u input; y output
function y = fcn(u)
y = length(u);
end
